simulink model "conical_tank"  (R2017b)
settings: Solver=VariableStepAuto  StartTime=0.0  StopTime=10000  MaxStep=0.1  RelTol=1e-3
settings Model: Creator=Laci  LastModifiedBy=Laci

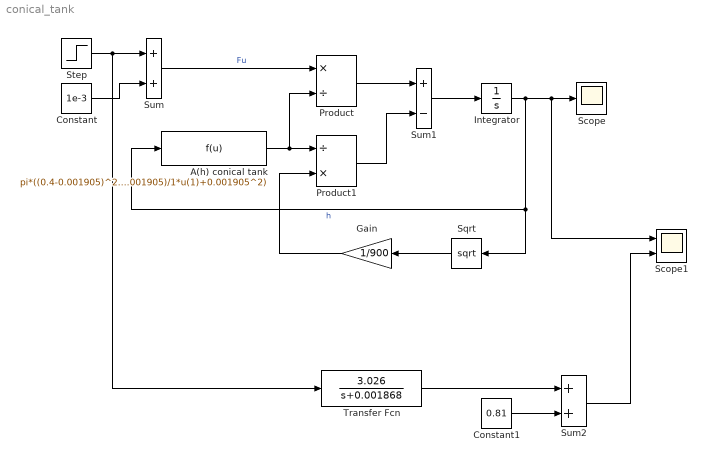
== system conical_tank ==
  A(h) conical tank : Fcn  Expr=pi*((0.4-0.001905)^2/1^2*u(1)^2+2*0.001905*(0.4-0.001905)/1*u(1)+0.001905^2)
  Constant : Constant  Value=1e-3
  Constant1 : Constant  Value=0.81
  Gain : Gain  Gain=1/900
  Integrator : Integrator  InitialCondition=1e-3
  Product : Product  Inputs=*/
  Product1 : Product  Inputs=/*
  Scope : Scope
  Scope1 : Scope  NumInputPorts=2
  Sqrt : Sqrt  SaturateOnIntegerOverflow=on
  Step : Step  Time=5000  After=1e-4  SampleTime=0
  Sum : Sum
  Sum1 : Sum  Inputs=+-
  Sum2 : Sum
  Transfer Fcn : TransferFcn  Numerator=[3.026]  Denominator=[1 0.001868]
  wires:
  Constant/1 -> Sum/2
  Sum/1 -> Product/1  "Fu"
  Product/1 -> Sum1/1
  Sum1/1 -> Integrator/1
  Integrator/1 -> Scope1/1, Scope/1, A(h) conical tank/1, Sqrt/1  "h"
  Sqrt/1 -> Gain/1
  Product1/1 -> Sum1/2
  Gain/1 -> Product1/2
  A(h) conical tank/1 -> Product/2, Product1/1
  Step/1 -> Transfer Fcn/1, Sum/1
  Constant1/1 -> Sum2/2
  Transfer Fcn/1 -> Sum2/1
  Sum2/1 -> Scope1/2
